simulink model "konstrukcijski_nadomjesne_direktni"  (R2018a)
settings: Solver=VariableStepAuto  StartTime=0.0  StopTime=10.0  RelTol=1e-3
libraries: simrfV2elements x23, simrfV2sources1 x6, simrfV2_lib x1
settings Model: Creator=Denis  LastModifiedBy=Denis

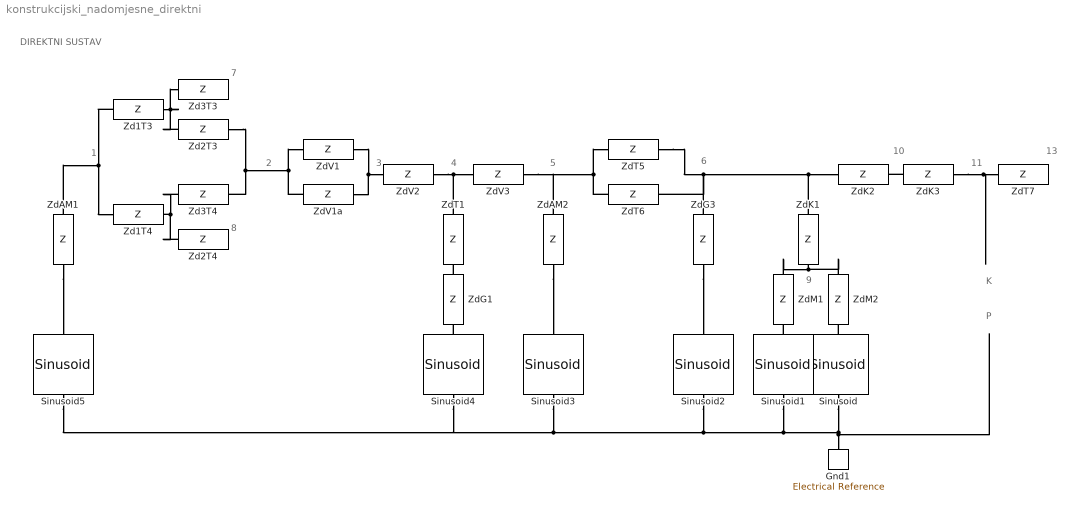
== system konstrukcijski_nadomjesne_direktni ==
  note: 13
  note: K
  note: DIREKTNI SUSTAV
  note: 11
  note: 10
  note: 9
  note: 6
  note: 5
  note: P
  note: 4
  note: 3
  note: 2
  note: 7
  note: 8
  note: 1
  Gnd1 : simrfV2_lib/Elements/Electrical Reference
  Sinusoid{,1..5} (6 alike) : simrfV2sources1/Sinusoid  SineSourceType=Ideal voltage  VO_I=0 V  IO_I=0 A  VO_Q=0 V  IO_Q=0 A  VA_I=0 V  IA_I=0 A  VA_Q=0 V  IA_Q=0 A  Fmod=0 Hz  TD=0 s  CarrierFreq=0 Hz  InternalGrounding=off
      settings: SourceProductName=RF Blockset  SourceProductBaseCode=RB
  Zd1T3 : simrfV2elements/Z  classname=complex_impedance  Impedance_type=Frequency independent  Impedance=50 + 30i  Freq=1e9 Hz
      settings: SourceProductName=RF Blockset  SourceProductBaseCode=RB
  Zd1T4 : simrfV2elements/Z  classname=complex_impedance  Impedance_type=Frequency independent  Impedance=50 + 30i  Freq=1e9 Hz
      settings: SourceProductName=RF Blockset  SourceProductBaseCode=RB
  Zd2T3 : simrfV2elements/Z  classname=complex_impedance  Impedance_type=Frequency independent  Impedance=50 + 30i  Freq=1e9 Hz
      settings: SourceProductName=RF Blockset  SourceProductBaseCode=RB
  Zd2T4 : simrfV2elements/Z  classname=complex_impedance  Impedance_type=Frequency independent  Impedance=50 + 30i  Freq=1e9 Hz
      settings: SourceProductName=RF Blockset  SourceProductBaseCode=RB
  Zd3T3 : simrfV2elements/Z  classname=complex_impedance  Impedance_type=Frequency independent  Impedance=50 + 30i  Freq=1e9 Hz
      settings: SourceProductName=RF Blockset  SourceProductBaseCode=RB
  Zd3T4 : simrfV2elements/Z  classname=complex_impedance  Impedance_type=Frequency independent  Impedance=50 + 30i  Freq=1e9 Hz
      settings: SourceProductName=RF Blockset  SourceProductBaseCode=RB
  ZdAM1 : simrfV2elements/Z  classname=complex_impedance  Impedance_type=Frequency independent  Impedance=50 + 30i  Freq=1e9 Hz
      settings: SourceProductName=RF Blockset  SourceProductBaseCode=RB
  ZdAM2 : simrfV2elements/Z  classname=complex_impedance  Impedance_type=Frequency independent  Impedance=50 + 30i  Freq=1e9 Hz
      settings: SourceProductName=RF Blockset  SourceProductBaseCode=RB
  ZdG1 : simrfV2elements/Z  classname=complex_impedance  Impedance_type=Frequency independent  Impedance=50 + 30i  Freq=1e9 Hz
      settings: SourceProductName=RF Blockset  SourceProductBaseCode=RB
  ZdG3 : simrfV2elements/Z  classname=complex_impedance  Impedance_type=Frequency independent  Impedance=50 + 30i  Freq=1e9 Hz
      settings: SourceProductName=RF Blockset  SourceProductBaseCode=RB
  ZdK1 : simrfV2elements/Z  classname=complex_impedance  Impedance_type=Frequency independent  Impedance=50 + 30i  Freq=1e9 Hz
      settings: SourceProductName=RF Blockset  SourceProductBaseCode=RB
  ZdK2 : simrfV2elements/Z  classname=complex_impedance  Impedance_type=Frequency independent  Impedance=50 + 30i  Freq=1e9 Hz
      settings: SourceProductName=RF Blockset  SourceProductBaseCode=RB
  ZdK3 : simrfV2elements/Z  classname=complex_impedance  Impedance_type=Frequency independent  Impedance=50 + 30i  Freq=1e9 Hz
      settings: SourceProductName=RF Blockset  SourceProductBaseCode=RB
  ZdM1 : simrfV2elements/Z  classname=complex_impedance  Impedance_type=Frequency independent  Impedance=50 + 30i  Freq=1e9 Hz
      settings: SourceProductName=RF Blockset  SourceProductBaseCode=RB
  ZdM2 : simrfV2elements/Z  classname=complex_impedance  Impedance_type=Frequency independent  Impedance=50 + 30i  Freq=1e9 Hz
      settings: SourceProductName=RF Blockset  SourceProductBaseCode=RB
  ZdT{1,5..7} (4 alike) : simrfV2elements/Z  classname=complex_impedance  Impedance_type=Frequency independent  Impedance=50 + 30i  Freq=1e9 Hz
      settings: SourceProductName=RF Blockset  SourceProductBaseCode=RB
  ZdV1 : simrfV2elements/Z  classname=complex_impedance  Impedance_type=Frequency independent  Impedance=50 + 30i  Freq=1e9 Hz
      settings: SourceProductName=RF Blockset  SourceProductBaseCode=RB
  ZdV1a : simrfV2elements/Z  classname=complex_impedance  Impedance_type=Frequency independent  Impedance=50 + 30i  Freq=1e9 Hz
      settings: SourceProductName=RF Blockset  SourceProductBaseCode=RB
  ZdV2 : simrfV2elements/Z  classname=complex_impedance  Impedance_type=Frequency independent  Impedance=50 + 30i  Freq=1e9 Hz
      settings: SourceProductName=RF Blockset  SourceProductBaseCode=RB
  ZdV3 : simrfV2elements/Z  classname=complex_impedance  Impedance_type=Frequency independent  Impedance=50 + 30i  Freq=1e9 Hz
      settings: SourceProductName=RF Blockset  SourceProductBaseCode=RB
  connections:
  ZdK3/LConn1 -- ZdK2/RConn1
  Gnd1/LConn1 -- Sinusoid5/RConn1 -- Sinusoid4/RConn1 -- Sinusoid3/RConn1 -- Sinusoid2/RConn1 -- Sinusoid1/RConn1 -- Sinusoid/RConn1
  Sinusoid/LConn1 -- ZdM2/RConn1
  Sinusoid1/LConn1 -- ZdM1/RConn1
  ZdM1/LConn1 -- ZdM2/LConn1 -- ZdK1/RConn1
  ZdG3/RConn1 -- Sinusoid2/LConn1
  ZdK1/LConn1 -- ZdT6/RConn1 -- ZdT5/RConn1 -- ZdG3/LConn1 -- ZdK2/LConn1
  ZdT6/LConn1 -- ZdAM2/LConn1 -- ZdV3/RConn1 -- ZdT5/LConn1
  ZdAM2/RConn1 -- Sinusoid3/LConn1
  ZdT1/LConn1 -- ZdV3/LConn1 -- ZdV2/RConn1
  ZdG1/LConn1 -- ZdT1/RConn1
  Sinusoid4/LConn1 -- ZdG1/RConn1
  ZdV1/RConn1 -- ZdV1a/RConn1 -- ZdV2/LConn1
  Zd2T3/RConn1 -- ZdV1/LConn1 -- ZdV1a/LConn1 -- Zd3T4/RConn1
  Zd1T3/RConn1 -- Zd2T3/LConn1 -- Zd3T3/LConn1
  Zd3T4/LConn1 -- Zd2T4/LConn1 -- Zd1T4/RConn1
  Zd1T3/LConn1 -- ZdAM1/LConn1 -- Zd1T4/LConn1
  ZdAM1/RConn1 -- Sinusoid5/LConn1
  ZdK3/RConn1 -- ZdT7/LConn1
